simulink model "pendulo"  (R2022a)
settings: Solver=ode4  StartTime=0.0  StopTime=800.0  FixedStep=0.01  RelTol=1e-3
settings Model: Creator=leonardonavacastellanos  LastModifiedBy=leonardonavacastellanos

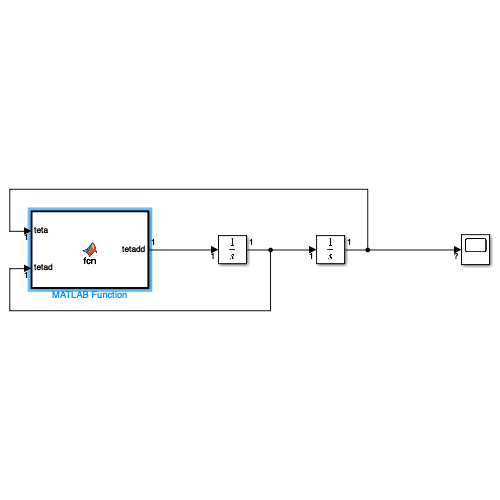
[thumbnail: Simulink's stored preview of the top-level diagram]
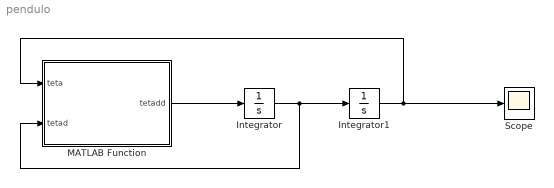
== system pendulo ==
  Integrator : Integrator
  Integrator1 : Integrator  InitialCondition=pi/2
  MATLAB Function : MATLAB Function  TreatAsAtomicUnit=on
  Scope : Scope
  wires:
  MATLAB Function/1(tetadd) -> Integrator/1
  Integrator/1 -> MATLAB Function/2(tetad), Integrator1/1
  Integrator1/1 -> Scope/1, MATLAB Function/1(teta)

== matlab function pendulo/MATLAB Function ==
  data: teta input; tetadd output; tetad input
function tetadd = fcn(teta,tetad)
K = 0.04;
m = 0.5;
l = 0.2;
g = 9.81;

tetadd = (1/m*l^2)*(-K*tetad - m*g*l*sin(teta));
